simulink model "Catalyst_Layer"  (R2016a)
settings: Solver=VariableStepAuto  StartTime=0.0  StopTime=10.0  RelTol=1e-3
settings Model: Creator=kwono  LastModifiedBy=kwono

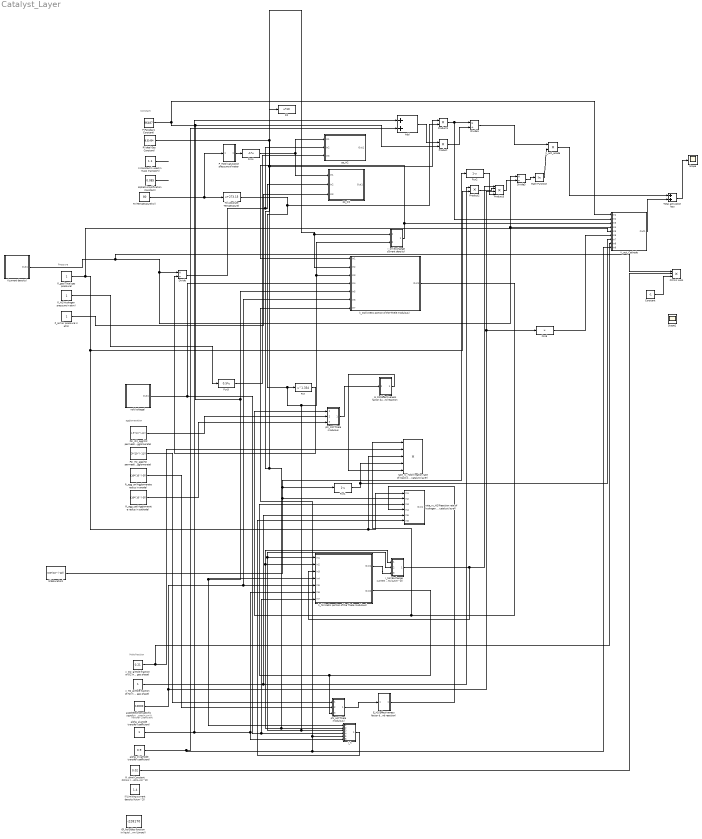
== system Catalyst_Layer ==
  note: Mole fraction
  note: Transfer Coefficient
  note: Pressure
  note: agglomeration
  note: Constant
  Add : Sum
  Constant : Constant  Value=-1
  Divide : Product  Inputs=*/
  Divide1 : Product  Inputs=*/
  Divide3 : Product  Inputs=*/
  E_H2(Effectiveness factor due to mass transfer and reaction) : Subsystem
  E_O2(Effectiveness factor due to mass transfer and reaction : Subsystem
  F(Faradays Constant) : Constant  Value=96487
  Fcn : Fcn  Expr=u^1.334
  Fcn1 : Fcn  Expr=1-u
  Fcn2 : Fcn  Expr=1-u
  Fcn3 : Fcn  Expr=0.5*u
  Fcn4 : Fcn  Expr=-1*u
  Fcn6 : Fcn  Expr=u
  Gf_liq(Gibbs function in liquid form (J/moe)) : Constant  Value=-228170
  Math Function : Math  Operator=log  SaturateOnIntegerOverflow=on
  Ohmic Loss : Product  Inputs=3
  P_H2(Hydrogen pressure in atm) : Constant
  P_H2O(saturation pressure of water : Subsystem
  P_air(air pressure in atm) : Constant
  P_gas(Total gas pressure) : Constant
  Product : Product
  Product1 : Product
  Product2 : Product
  Product3 : Product  Inputs=4
  Psi_H2_agg(H2 permeation in agglomerate) : Constant  Value=2*(10^(-11))
  Psi_O2_agg(O2 permeation in agglomerate) : Constant  Value=1.5*(10^(-11))
  R(Ideal Gas Constant) : Constant  Value=8.31434
  R2 : Fcn  Expr=u*10
  R_agg_an(Agglomerate radius in anode) : Constant  Value=110*(10^(-5))
  R_agg_cat(Agglomerate radius in cathode) : Constant  Value=110*(10^(-5))
  R_ohm(Constant Ohmic resistance(ohm-cm^2)) : Constant  Value=0.02
  S(Saturation) : Constant  Value=0.6*(10^(-12))
  Scope : Scope
  Scope1 : Scope
  Tc(Temperature(C)) : Constant  Value=80
  Tk(Absolute Temperature) : Fcn  Expr=u+273.15
  Total activation loss : Sum
  V_act_Cathode : Subsystem
  V_act_anode : Product
  a120(Electroe specific interfacial area(1/cm)) : Constant  Value=10000
  alpha1(Amplification Constant) : Constant  Value=0.085
  alpha_a(anode transfer coefficient) : Constant
  alpha_c(cathode transfer coefficient) : Constant  Value=0.9
  i(current density) : Subsystem
  i_h : Subsystem
  i_hor(Exchange current density(A/cm^2)) : Subsystem
  i_orr(exchange current density) : Subsystem
  il(Limiting current density(A/cm^2)) : Constant  Value=1.4
  k(constant k used in mass transport) : Constant  Value=1.1
  k_O2(kinetic portion of the Thiele modulous) : Subsystem
  k_h(Kinetic portion of the Thiele modulous) : Subsystem
  phi_H2(Thiele modulous) : Subsystem
  phi_O2(Thiele modulous : Subsystem
  pp_H2 : Subsystem
  pp_O2 : Subsystem
  rate_rx_H2(Reaction rate of hydrogen at anode catalyst layer) : Subsystem
  rate_rx_H2Ol(reation rate of liquid water at cathode catalyst layer) : Product  Inputs=5
  volt(voltage) : Subsystem
  x_H2_g(Mole fraction of H2 in the gas phase) : Constant
  x_O2_g(Mole fraction of O2 in the gas phase) : Constant  Value=0.21
  wires:
  Tc(Temperature(C))/1 -> Tk(Absolute Temperature)/1, P_H2O(saturation pressure of water/1(In1)
  Fcn/1 -> Divide/2
  P_H2O(saturation pressure of water/1(Out1) -> Fcn4/1
  P_H2(Hydrogen pressure in atm)/1 -> Fcn3/1
  P_air(air pressure in atm)/1 -> pp_O2/3(In3)
  i(current density)/1(Out1) -> Ohmic Loss/1, Divide3/1, V_act_Cathode/4(In4), Divide/1
  Divide/1 -> pp_O2/2(In2), pp_H2/2(In2)
  Fcn4/1 -> pp_O2/1(In1), pp_H2/1(In1)
  Fcn3/1 -> pp_H2/3(In3)
  k(constant k used in mass transport)/1 -> ?
  alpha1(Amplification Constant)/1 -> ?
  Psi_O2_agg(O2 permeation in agglomerate)/1 -> phi_O2(Thiele modulous/2(In2)
  R_agg_cat(Agglomerate radius in cathode)/1 -> phi_O2(Thiele modulous/3(In3)
  phi_O2(Thiele modulous/1(Out1) -> E_O2(Effectiveness factor due to mass transfer and reaction/1(In1)
  S(Saturation)/1 -> rate_rx_H2(Reaction rate of hydrogen at anode catalyst layer)/2(In2), Fcn2/1, Fcn1/1
  P_gas(Total gas pressure)/1 -> V_act_Cathode/5(In5), Product2/2, rate_rx_H2(Reaction rate of hydrogen at anode catalyst layer)/1(In1), rate_rx_H2Ol(reation rate of liquid water at cathode catalyst layer)/3
  Fcn1/1 -> rate_rx_H2Ol(reation rate of liquid water at cathode catalyst layer)/4, V_act_Cathode/7(In7)
  E_O2(Effectiveness factor due to mass transfer and reaction/1(Out1) -> rate_rx_H2Ol(reation rate of liquid water at cathode catalyst layer)/5
  x_O2_g(Mole fraction of O2 in the gas phase)/1 -> V_act_Cathode/8(In8), rate_rx_H2Ol(reation rate of liquid water at cathode catalyst layer)/2
  Psi_H2_agg(H2 permeation in agglomerate)/1 -> phi_H2(Thiele modulous)/1(In1)
  R_agg_an(Agglomerate radius in anode)/1 -> phi_H2(Thiele modulous)/2(In2)
  phi_H2(Thiele modulous)/1(Out1) -> E_H2(Effectiveness factor due to mass transfer and reaction)/1(In1)
  E_H2(Effectiveness factor due to mass transfer and reaction)/1(Out1) -> rate_rx_H2(Reaction rate of hydrogen at anode catalyst layer)/4(In4)
  x_H2_g(Mole fraction of H2 in the gas phase)/1 -> Product2/1, rate_rx_H2(Reaction rate of hydrogen at anode catalyst layer)/5(In5)
  i_h/1(Out1) -> rate_rx_H2(Reaction rate of hydrogen at anode catalyst layer)/6(In6)
  Add/1 -> Product/1
  Product1/1 -> V_act_Cathode/2(In2), Divide1/1
  Product/1 -> Divide1/2
  alpha_a(anode transfer coefficient)/1 -> Add/1, k_h(Kinetic portion of the Thiele modulous)/6(In6), i_h/6(In6)
  k_h(Kinetic portion of the Thiele modulous)/2(Out2) -> rate_rx_H2(Reaction rate of hydrogen at anode catalyst layer)/3(In3), phi_H2(Thiele modulous)/3(In3)
  i_hor(Exchange current density(A/cm^2))/1(Out1) -> Product3/1, k_h(Kinetic portion of the Thiele modulous)/3(In3)
  k_h(Kinetic portion of the Thiele modulous)/1(Out1) -> i_hor(Exchange current density(A/cm^2))/3(In3)
  Product2/1 -> Product3/2
  Fcn2/1 -> Product3/4
  Product3/1 -> Divide3/2
  Divide3/1 -> Math Function/1
  Divide1/1 -> V_act_anode/1
  Math Function/1 -> V_act_anode/2
  volt(voltage)/1(Out1) -> k_O2(kinetic portion of the Thiele modulous)/4(In4), i_h/4(In4), k_h(Kinetic portion of the Thiele modulous)/7(In7)
  a120(Electroe specific interfacial area(1/cm))/1 -> Fcn6/1, Product3/3, k_O2(kinetic portion of the Thiele modulous)/6(In6), k_h(Kinetic portion of the Thiele modulous)/5(In5)
  alpha_c(cathode transfer coefficient)/1 -> V_act_Cathode/9(In9), k_O2(kinetic portion of the Thiele modulous)/7(In7), i_h/5(In5), Add/2
  F(Faradays Constant)/1 -> V_act_Cathode/1(In1), Product/2, k_O2(kinetic portion of the Thiele modulous)/5(In5), i_h/1(In1), k_h(Kinetic portion of the Thiele modulous)/4(In4)
  R(Ideal Gas Constant)/1 -> Product1/1, i_hor(Exchange current density(A/cm^2))/1(In1), k_h(Kinetic portion of the Thiele modulous)/2(In2), i_h/2(In2), i_orr(exchange current density)/1(In1), k_O2(kinetic portion of the Thiele modulous)/2(In2), R2/1
  Tk(Absolute Temperature)/1 -> Product1/2, i_orr(exchange current density)/2(In2), k_O2(kinetic portion of the Thiele modulous)/3(In3), i_hor(Exchange current density(A/cm^2))/2(In2), k_h(Kinetic portion of the Thiele modulous)/1(In1), i_h/3(In3), Fcn/1
  k_O2(kinetic portion of the Thiele modulous)/1(Out1) -> phi_O2(Thiele modulous/1(In1), rate_rx_H2Ol(reation rate of liquid water at cathode catalyst layer)/1
  i_orr(exchange current density)/1(Out1) -> k_O2(kinetic portion of the Thiele modulous)/1(In1), V_act_Cathode/3(In3)
  V_act_anode/1 -> Total activation loss/1
  Total activation loss/1 -> Scope/1
  Fcn6/1 -> V_act_Cathode/6(In6)
  V_act_Cathode/1(Out1) -> Total activation loss/2
  R_ohm(Constant Ohmic resistance(ohm-cm^2))/1 -> Ohmic Loss/2
  Constant/1 -> Ohmic Loss/3

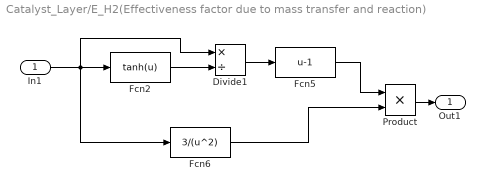
== system Catalyst_Layer/E_H2(Effectiveness factor due to mass transfer and reaction) ==
  In1 : Inport
  Divide1 : Product  Inputs=*/
  Fcn2 : Fcn  Expr=tanh(u)
  Fcn5 : Fcn  Expr=u-1
  Fcn6 : Fcn  Expr=3/(u^2)
  Product : Product
  Out1 : Outport
  wires:
  Fcn5/1 -> Product/1
  Fcn2/1 -> Divide1/2
  Divide1/1 -> Fcn5/1
  In1/1 -> Fcn2/1, Fcn6/1, Divide1/1
  Fcn6/1 -> Product/2
  Product/1 -> Out1/1

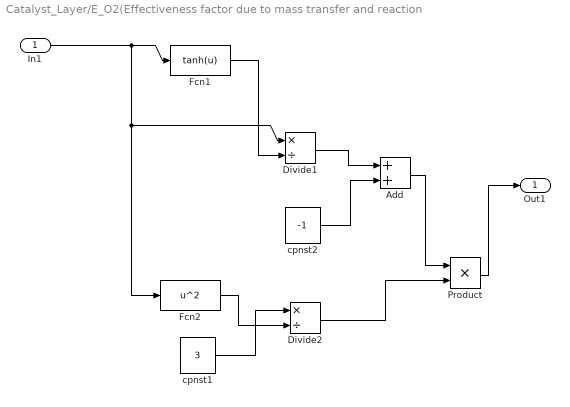
== system Catalyst_Layer/E_O2(Effectiveness factor due to mass transfer and reaction ==
  In1 : Inport
  Add : Sum
  Divide1 : Product  Inputs=*/
  Divide2 : Product  Inputs=*/
  Fcn1 : Fcn  Expr=tanh(u)
  Fcn2 : Fcn  Expr=u^2
  Product : Product
  cpnst1 : Constant  Value=3
  cpnst2 : Constant  Value=-1
  Out1 : Outport
  wires:
  Add/1 -> Product/1
  cpnst2/1 -> Add/2
  In1/1 -> Fcn2/1, Divide1/1, Fcn1/1
  Fcn2/1 -> Divide2/2
  Divide2/1 -> Product/2
  cpnst1/1 -> Divide2/1
  Fcn1/1 -> Divide1/2
  Divide1/1 -> Add/1
  Product/1 -> Out1/1

== system Catalyst_Layer/P_H2O(saturation pressure of water ==
  In1 : Inport
  Math Function : Math  Operator=10^u  SaturateOnIntegerOverflow=on
  x : Subsystem
  Out1 : Outport
  wires:
  x/1(Out1) -> Math Function/1
  In1/1 -> x/1(In1)
  Math Function/1 -> Out1/1

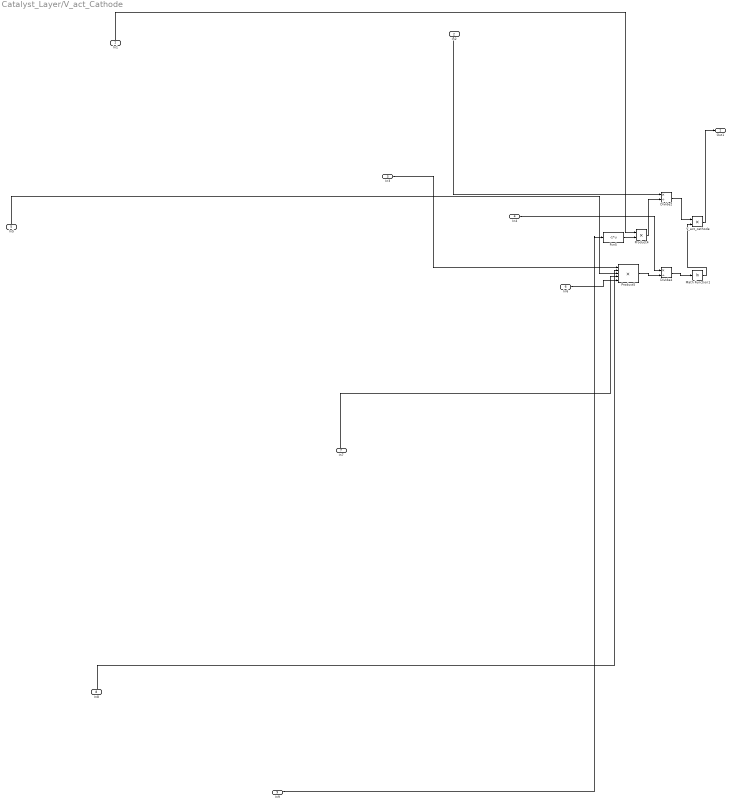
== system Catalyst_Layer/V_act_Cathode ==
  In1 : Inport
  In2 : Inport  Port=2
  In3 : Inport  Port=3
  In4 : Inport  Port=4
  In5 : Inport  Port=5
  In6 : Inport  Port=6
  In7 : Inport  Port=7
  In8 : Inport  Port=8
  In9 : Inport  Port=9
  Divide2 : Product  Inputs=*/
  Divide4 : Product  Inputs=*/
  Fcn5 : Fcn  Expr=-1*u
  Math Function1 : Math  Operator=log  SaturateOnIntegerOverflow=on
  Product4 : Product
  Product5 : Product  Inputs=5
  V_act_cathode : Product
  Out1 : Outport
  wires:
  Product4/1 -> Divide2/2
  Fcn5/1 -> Product4/2
  In6/1 -> Product5/5
  Product5/1 -> Divide4/2
  Divide4/1 -> Math Function1/1
  In8/1 -> Product5/2
  In2/1 -> Divide2/1
  In5/1 -> Product5/3
  In3/1 -> Product5/1
  In4/1 -> Divide4/1
  In1/1 -> Product4/1
  In7/1 -> Product5/4
  In9/1 -> Fcn5/1
  Math Function1/1 -> V_act_cathode/2
  V_act_cathode/1 -> Out1/1
  Divide2/1 -> V_act_cathode/1

== system Catalyst_Layer/i(current density) ==
  Add : Sum
  Constant1 : Constant  Value=0.01
  Delay : Delay  DelayLength=1  InitialCondition=0  SampleTime=0.01
  Out1 : Outport
  wires:
  Constant1/1 -> Add/1
  Delay/1 -> Add/2
  Add/1 -> Out1/1, Delay/1

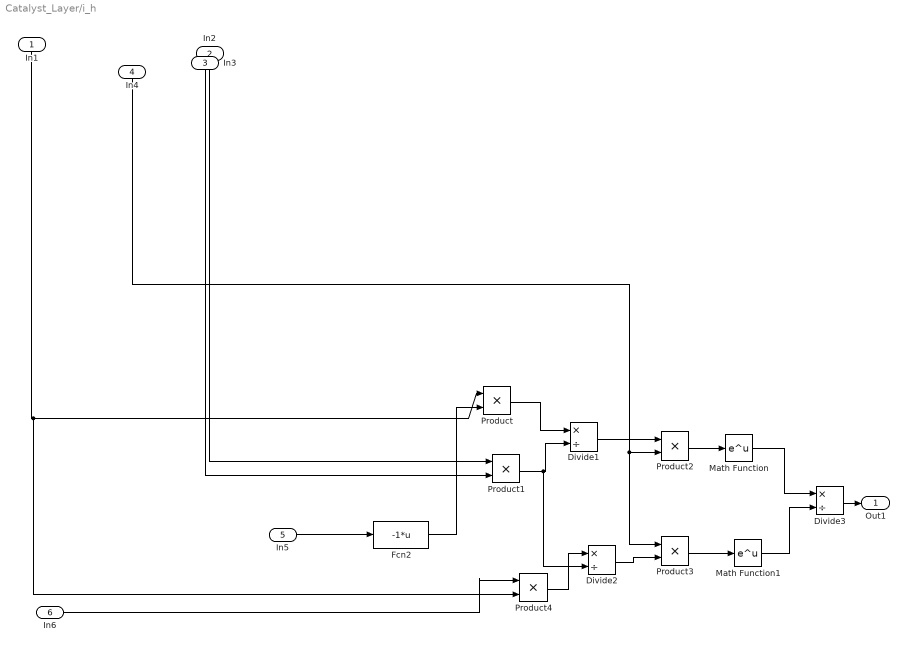
== system Catalyst_Layer/i_h ==
  In1 : Inport
  In2 : Inport  Port=2
  In3 : Inport  Port=3
  In4 : Inport  Port=4
  In5 : Inport  Port=5
  In6 : Inport  Port=6
  Divide1 : Product  Inputs=*/
  Divide2 : Product  Inputs=*/
  Divide3 : Product  Inputs=*/
  Fcn2 : Fcn  Expr=-1*u
  Math Function : Math  SaturateOnIntegerOverflow=on
  Math Function1 : Math  SaturateOnIntegerOverflow=on
  Product{,1..4} (5 alike) : Product
  Out1 : Outport
  wires:
  Product1/1 -> Divide2/2, Divide1/2
  Math Function1/1 -> Divide3/2
  Product3/1 -> Math Function1/1
  Fcn2/1 -> Product/2
  Math Function/1 -> Divide3/1
  Product4/1 -> Divide2/1
  In3/1 -> Product1/2
  In2/1 -> Product1/1
  Divide3/1 -> Out1/1
  In4/1 -> Product2/2, Product3/1
  In5/1 -> Fcn2/1
  In1/1 -> Product4/2, Product/1
  In6/1 -> Product4/1
  Divide2/1 -> Product3/2
  Divide1/1 -> Product2/1
  Product2/1 -> Math Function/1
  Product/1 -> Divide1/1

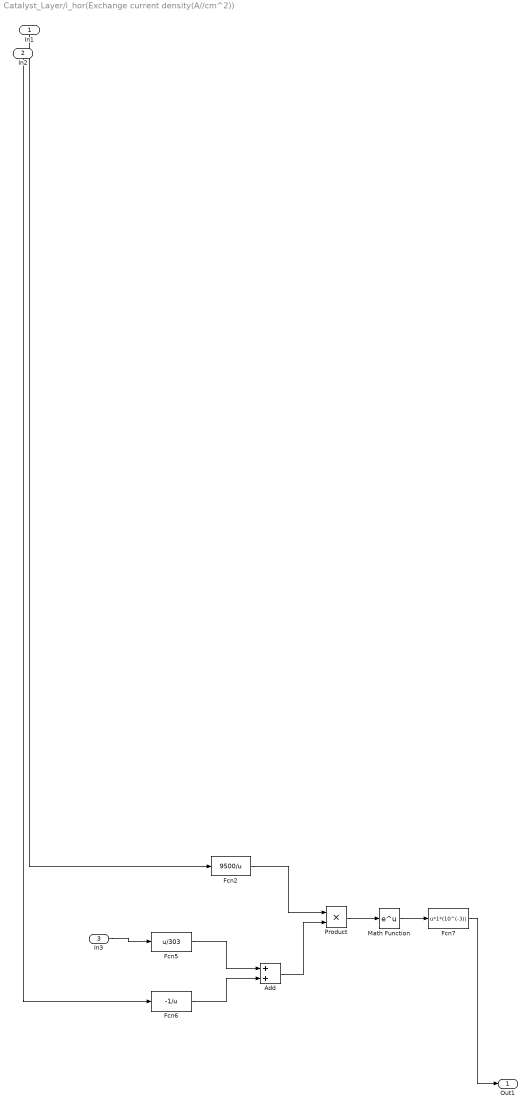
== system Catalyst_Layer/i_hor(Exchange current density(A//cm^2)) ==
  In1 : Inport
  In2 : Inport  Port=2
  In3 : Inport  Port=3
  Add : Sum
  Fcn2 : Fcn  Expr=9500/u
  Fcn5 : Fcn  Expr=u/303
  Fcn6 : Fcn  Expr=-1/u
  Fcn7 : Fcn  Expr=u*1*(10^(-3))
  Math Function : Math  SaturateOnIntegerOverflow=on
  Product : Product
  Out1 : Outport
  wires:
  Math Function/1 -> Fcn7/1
  Fcn5/1 -> Add/1
  Fcn6/1 -> Add/2
  Fcn7/1 -> Out1/1
  In3/1 -> Fcn5/1
  In2/1 -> Fcn6/1
  In1/1 -> Fcn2/1
  Add/1 -> Product/2
  Product/1 -> Math Function/1
  Fcn2/1 -> Product/1

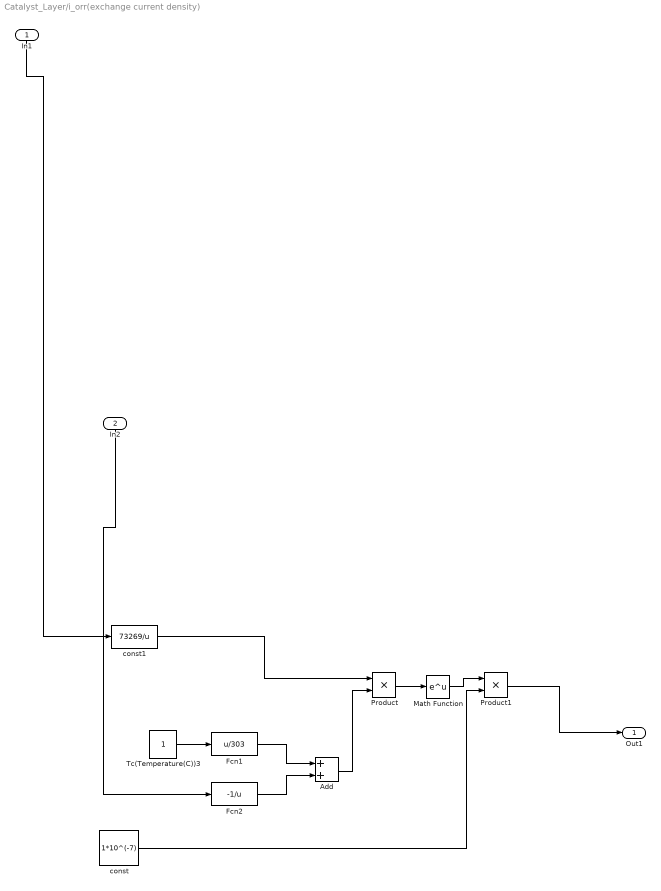
== system Catalyst_Layer/i_orr(exchange current density) ==
  In1 : Inport
  In2 : Inport  Port=2
  Add : Sum
  Fcn1 : Fcn  Expr=u/303
  Fcn2 : Fcn  Expr=-1/u
  Math Function : Math  SaturateOnIntegerOverflow=on
  Product : Product
  Product1 : Product
  Tc(Temperature(C))3 : Constant
  const : Constant  Value=1*10^(-7)
  const1 : Fcn  Expr=73269/u
  Out1 : Outport
  wires:
  Math Function/1 -> Product1/1
  const1/1 -> Product/1
  Tc(Temperature(C))3/1 -> Fcn1/1
  Product/1 -> Math Function/1
  Add/1 -> Product/2
  Fcn2/1 -> Add/2
  In2/1 -> Fcn2/1
  In1/1 -> const1/1
  const/1 -> Product1/2
  Product1/1 -> Out1/1
  Fcn1/1 -> Add/1

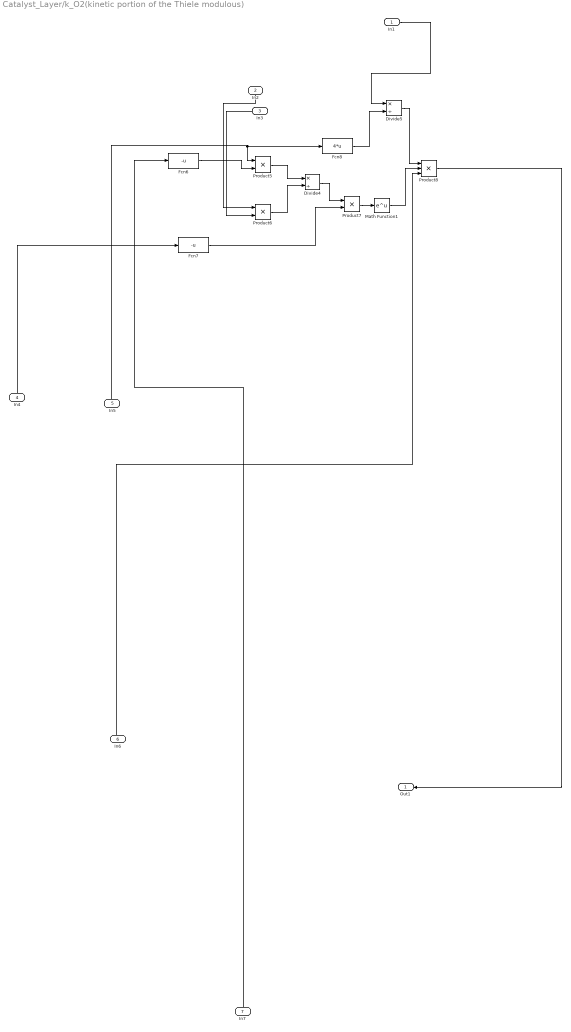
== system Catalyst_Layer/k_O2(kinetic portion of the Thiele modulous) ==
  In1 : Inport
  In2 : Inport  Port=2
  In3 : Inport  Port=3
  In4 : Inport  Port=4
  In5 : Inport  Port=5
  In6 : Inport  Port=6
  In7 : Inport  Port=7
  Divide4 : Product  Inputs=*/
  Divide5 : Product  Inputs=*/
  Fcn6 : Fcn  Expr=-u
  Fcn7 : Fcn  Expr=-u
  Fcn8 : Fcn  Expr=4*u
  Math Function1 : Math  SaturateOnIntegerOverflow=on
  Product5 : Product
  Product6 : Product
  Product7 : Product
  Product8 : Product  Inputs=3
  Out1 : Outport
  wires:
  In6/1 -> Product8/3
  In7/1 -> Fcn6/1
  In5/1 -> Fcn8/1, Product5/1
  In3/1 -> Product6/2
  In2/1 -> Product6/1
  In4/1 -> Fcn7/1
  Product5/1 -> Divide4/1
  Fcn7/1 -> Product7/2
  Fcn8/1 -> Divide5/2
  Divide4/1 -> Product7/1
  Fcn6/1 -> Product5/2
  Product6/1 -> Divide4/2
  Product7/1 -> Math Function1/1
  Divide5/1 -> Product8/1
  In1/1 -> Divide5/1
  Math Function1/1 -> Product8/2
  Product8/1 -> Out1/1

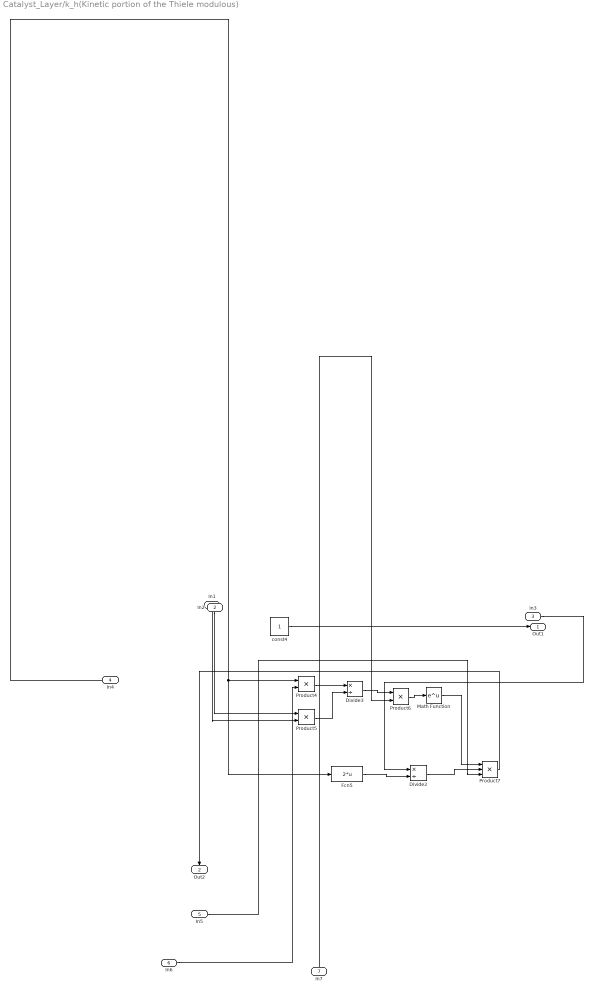
== system Catalyst_Layer/k_h(Kinetic portion of the Thiele modulous) ==
  In1 : Inport
  In2 : Inport  Port=2
  In3 : Inport  Port=3
  In4 : Inport  Port=4
  In5 : Inport  Port=5
  In6 : Inport  Port=6
  In7 : Inport  Port=7
  Divide2 : Product  Inputs=*/
  Divide3 : Product  Inputs=*/
  Fcn5 : Fcn  Expr=2*u
  Math Function : Math  SaturateOnIntegerOverflow=on
  Product4 : Product
  Product5 : Product
  Product6 : Product
  Product7 : Product  Inputs=3
  const4 : Constant
  Out1 : Outport
  Out2 : Outport  Port=2
  wires:
  Product7/1 -> Out2/1
  Math Function/1 -> Product7/1
  Fcn5/1 -> Divide2/2
  const4/1 -> Out1/1
  Product5/1 -> Divide3/2
  Product4/1 -> Divide3/1
  Divide3/1 -> Product6/1
  In3/1 -> Divide2/1
  Divide2/1 -> Product7/2
  Product6/1 -> Math Function/1
  In5/1 -> Product7/3
  In4/1 -> Fcn5/1, Product4/1
  In2/1 -> Product5/1
  In6/1 -> Product4/2
  In1/1 -> Product5/2
  In7/1 -> Product6/2

== system Catalyst_Layer/phi_H2(Thiele modulous) ==
  In1 : Inport
  In2 : Inport  Port=2
  In3 : Inport  Port=3
  Divide1 : Product  Inputs=*/
  Fcn2 : Fcn  Expr=u^(0.5)
  Product : Product
  Out1 : Outport
  wires:
  Product/1 -> Out1/1
  In1/1 -> Divide1/2
  In2/1 -> Product/1
  In3/1 -> Divide1/1
  Divide1/1 -> Fcn2/1
  Fcn2/1 -> Product/2

== system Catalyst_Layer/phi_O2(Thiele modulous ==
  In1 : Inport
  In2 : Inport  Port=2
  In3 : Inport  Port=3
  Divide1 : Product  Inputs=*/
  Fcn1 : Fcn  Expr=u^(0.5)
  Product : Product
  Out1 : Outport
  wires:
  In1/1 -> Divide1/1
  Product/1 -> Out1/1
  In2/1 -> Divide1/2
  In3/1 -> Product/2
  Divide1/1 -> Fcn1/1
  Fcn1/1 -> Product/1

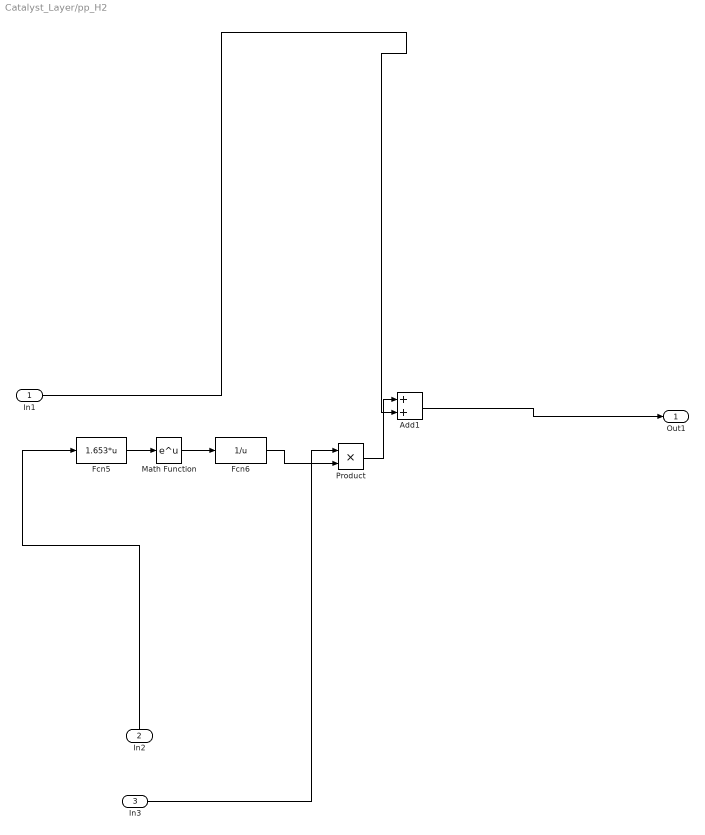
== system Catalyst_Layer/pp_H2 ==
  In1 : Inport
  In2 : Inport  Port=2
  In3 : Inport  Port=3
  Add1 : Sum
  Fcn5 : Fcn  Expr=1.653*u
  Fcn6 : Fcn  Expr=1/u
  Math Function : Math  SaturateOnIntegerOverflow=on
  Product : Product
  Out1 : Outport
  wires:
  In1/1 -> Add1/2
  In2/1 -> Fcn5/1
  Add1/1 -> Out1/1
  Fcn6/1 -> Product/2
  Fcn5/1 -> Math Function/1
  In3/1 -> Product/1
  Product/1 -> Add1/1
  Math Function/1 -> Fcn6/1

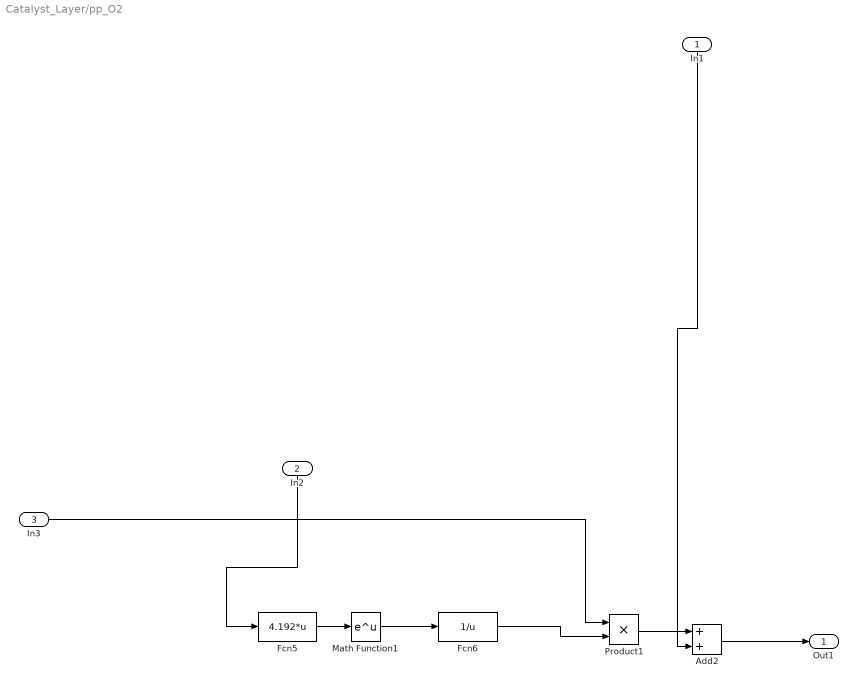
== system Catalyst_Layer/pp_O2 ==
  In1 : Inport
  In2 : Inport  Port=2
  In3 : Inport  Port=3
  Add2 : Sum
  Fcn5 : Fcn  Expr=4.192*u
  Fcn6 : Fcn  Expr=1/u
  Math Function1 : Math  SaturateOnIntegerOverflow=on
  Product1 : Product
  Out1 : Outport
  wires:
  Math Function1/1 -> Fcn6/1
  Fcn5/1 -> Math Function1/1
  Fcn6/1 -> Product1/2
  In1/1 -> Add2/2
  In2/1 -> Fcn5/1
  In3/1 -> Product1/1
  Product1/1 -> Add2/1
  Add2/1 -> Out1/1

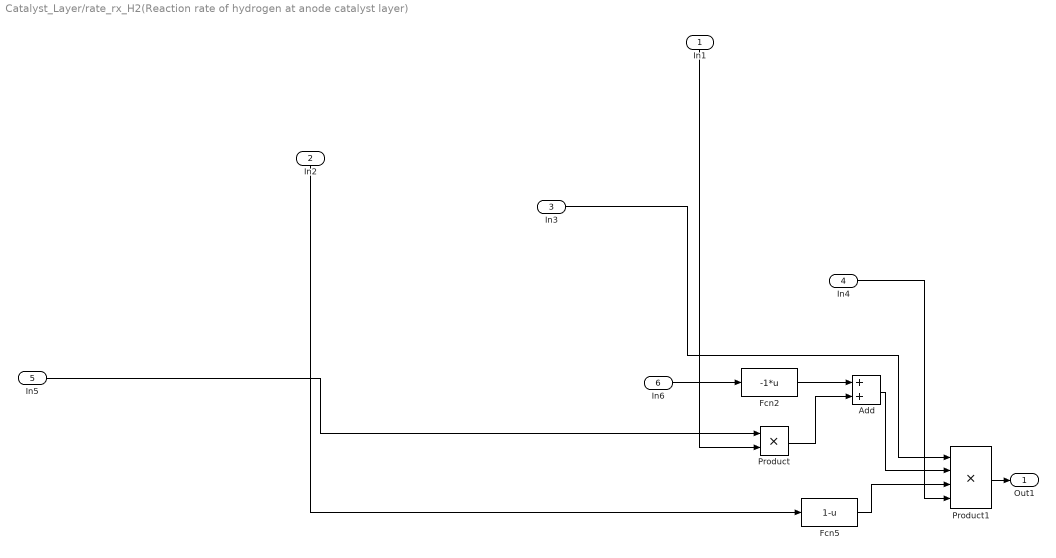
== system Catalyst_Layer/rate_rx_H2(Reaction rate of hydrogen at anode catalyst layer) ==
  In1 : Inport
  In2 : Inport  Port=2
  In3 : Inport  Port=3
  In4 : Inport  Port=4
  In5 : Inport  Port=5
  In6 : Inport  Port=6
  Add : Sum
  Fcn2 : Fcn  Expr=-1*u
  Fcn5 : Fcn  Expr=1-u
  Product : Product
  Product1 : Product  Inputs=4
  Out1 : Outport
  wires:
  Add/1 -> Product1/2
  In3/1 -> Product1/1
  In2/1 -> Fcn5/1
  In1/1 -> Product/2
  Product1/1 -> Out1/1
  In5/1 -> Product/1
  Fcn2/1 -> Add/1
  Product/1 -> Add/2
  In6/1 -> Fcn2/1
  In4/1 -> Product1/4
  Fcn5/1 -> Product1/3

== system Catalyst_Layer/volt(voltage) ==
  Add : Sum
  Constant1 : Constant  Value=0.01
  Delay : Delay  DelayLength=1  InitialCondition=0  SampleTime=0.01
  Out1 : Outport
  wires:
  Constant1/1 -> Add/1
  Delay/1 -> Add/2
  Add/1 -> Out1/1, Delay/1

== system Catalyst_Layer/P_H2O(saturation pressure of water/x ==
  In1 : Inport
  Add : Sum  Inputs=++++
  Constant1 : Constant  Value=-2.1794
  R1 : Fcn  Expr=0.02953*u
  R3 : Fcn  Expr=-9.1837*(10^(-5))*(u^2)
  R4 : Fcn  Expr=1.4454*(10^(-7))*(u^3)
  Out1 : Outport
  wires:
  In1/1 -> R4/1, R3/1, R1/1
  Constant1/1 -> Add/1
  R4/1 -> Add/4
  Add/1 -> Out1/1
  R1/1 -> Add/2
  R3/1 -> Add/3
